simulink model "ShaftSensor"  (R2014a)
settings: Solver=ode45  StartTime=0.0  StopTime=10.0  RelTol=1e-3
values from neighbouring files (symbols this model uses):
  SampleTime = 0.01    [Lab_6_01.m]
settings Model: Creator=williamsd  LastModifiedBy=williamsd

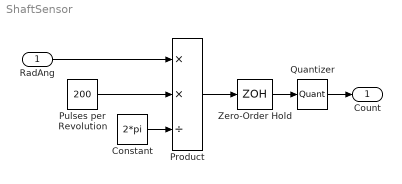
== system ShaftSensor ==
  RadAng : Inport
  Constant : Constant  Value=2*pi
  Product : Product  Inputs=**/
  "Pulses per Revolution " : Constant  Value=200
  Quantizer : Quantizer  QuantizationInterval=1
  Zero-Order Hold : ZeroOrderHold  SampleTime=SampleTime
  Count : Outport
  wires:
  "Pulses per Revolution "/1 -> Product/2
  Constant/1 -> Product/3
  RadAng/1 -> Product/1
  Product/1 -> Zero-Order Hold/1
  Zero-Order Hold/1 -> Quantizer/1
  Quantizer/1 -> Count/1
